simulink model "ALL_JP360_DBW_V6_5_1103"  (R2022a)
settings: Solver=FixedStepAuto  StartTime=0.0  StopTime=inf  FixedStep=0.01  RelTol=1e-3  EnableMultiTasking=on
model workspace (MAT data in the model file):
  g = 9.8
undefined symbols (not defined in the file or in its folder): canChannel, delta_v_p, IPM_Line_C0, IPM_Line_C1, IPM_Line_C2, IPM_Line_C3, M, M_p, MRR_ObjDistX, MRR_ObjDistY, MRR_ObjFusionCamID, MRR_ObjFusionSig, MRR_ObjID, MRR_ObjRelVelX, MRR_ObjRelVelY, MRR_ObjType, MRR_ObjUpdFlg, none, obj_vaild, untracktime, V, videoinput
libraries: canfdmsglib x230, canfdlib x76, slpidlib x24, simulink x18, dspstat3 x14, ctrlSharedLib x1, simulink_extras x1, imaqlib x1, realtime_pacer_lib x1, dspvision x1, visionsinks x1
(part 3 of 55)

== system ALL_JP360_DBW_V6_5_1103/MsgToCAN ==
  ACC_Torque_Request : Inport
  ACC_Torque_Request_Status : Inport  Port=2
  ACC_TgtAx : Inport  Port=3
  ACC_BrakePreferred : Inport  Port=4
  ACC_StandstillReq : Inport  Port=5
  ACC_Status : Inport  Port=6
  setvspped : Inport  Port=7
  ACC_TimeGapSet : Inport  Port=8
  ACC_EngineStartstop : Inport  Port=9
  IPM_LaneAssit_Status : Inport  Port=10
  IPM_LaneAssit_TorqueReq : Inport  Port=11
  IPM_LaneAssit_TorqueReqStatus : Inport  Port=12
  Obj_Speed : Inport  Port=13
  ACC_ObjDetected : Inport  Port=14
  MRR_L_Obj_0x_class : Inport  Port=15
  MRR_L_Object_dx : Inport  Port=16
  MRR_L_Object_dy : Inport  Port=17
  MRR_LeftTargetDetection : Inport  Port=18
  MRR_R_Obj_0x_class : Inport  Port=19
  MRR_R_Object_dx : Inport  Port=20
  MRR_R_Object_dy : Inport  Port=21
  MRR_RightTargetDetection : Inport  Port=22
  MRR_F_Object_dx : Inport  Port=23
  MRR_F_Object_dy : Inport  Port=24
  MRR_F_Obj_0x_class : Inport  Port=25
  640 : Inport  Port=26
  641 : Inport  Port=27
  642 : Inport  Port=28
  643 : Inport  Port=29
  ACC_DriveOff : Inport  Port=30
  CAN FD Transmit1 : canfdlib/CAN FD Transmit  BlockHandle=28204.001  Device=Vector VN1640A 1 (Channel 3)  ObjConstructor=canChannel('Vector', 'VN1640A 1', 3, 'ProtocolMode', 'CAN FD')  EnableEventTransmit=off  EnablePeriodicTransmit=on  MessagePeriod=0.02
      settings: SourceProductBaseCode=VN
  CAN FD Transmit10 : canfdlib/CAN FD Transmit  BlockHandle=28206.001  Device=Vector VN1640A 1 (Channel 3)  ObjConstructor=canChannel('Vector', 'VN1640A 1', 3, 'ProtocolMode', 'CAN FD')  EnableEventTransmit=off  EnablePeriodicTransmit=on  MessagePeriod=0.1
      settings: SourceProductBaseCode=VN
  CAN FD Transmit11 : canfdlib/CAN FD Transmit  BlockHandle=28208.001  Device=Vector VN1640A 1 (Channel 3)  ObjConstructor=canChannel('Vector', 'VN1640A 1', 3, 'ProtocolMode', 'CAN FD')  EnableEventTransmit=off  EnablePeriodicTransmit=on  MessagePeriod=0.1
      settings: SourceProductBaseCode=VN
  CAN FD Transmit2 : canfdlib/CAN FD Transmit  BlockHandle=28210.001  Device=Vector VN1640A 1 (Channel 3)  ObjConstructor=canChannel('Vector', 'VN1640A 1', 3, 'ProtocolMode', 'CAN FD')  EnableEventTransmit=off  EnablePeriodicTransmit=on  MessagePeriod=0.02
      settings: SourceProductBaseCode=VN
  CAN FD Transmit3 : canfdlib/CAN FD Transmit  BlockHandle=28212.001  Device=Vector VN1640A 1 (Channel 3)  ObjConstructor=canChannel('Vector', 'VN1640A 1', 3, 'ProtocolMode', 'CAN FD')  EnableEventTransmit=off  EnablePeriodicTransmit=on  MessagePeriod=0.02
      settings: SourceProductBaseCode=VN
  CAN FD Transmit4 : canfdlib/CAN FD Transmit  BlockHandle=28214.001  Device=Vector VN1640A 1 (Channel 3)  ObjConstructor=canChannel('Vector', 'VN1640A 1', 3, 'ProtocolMode', 'CAN FD')  EnableEventTransmit=off  EnablePeriodicTransmit=on  MessagePeriod=0.02
      settings: SourceProductBaseCode=VN
  CAN FD Transmit5 : canfdlib/CAN FD Transmit  BlockHandle=28216.001  Device=Vector VN1640A 1 (Channel 3)  ObjConstructor=canChannel('Vector', 'VN1640A 1', 3, 'ProtocolMode', 'CAN FD')  EnableEventTransmit=off  EnablePeriodicTransmit=on  MessagePeriod=0.02
      settings: SourceProductBaseCode=VN
  CAN FD Transmit6 : canfdlib/CAN FD Transmit  BlockHandle=28218.001  Device=Vector VN1640A 1 (Channel 3)  ObjConstructor=canChannel('Vector', 'VN1640A 1', 3, 'ProtocolMode', 'CAN FD')  EnableEventTransmit=off  EnablePeriodicTransmit=on  MessagePeriod=0.02
      settings: SourceProductBaseCode=VN
  CAN FD Transmit7 : canfdlib/CAN FD Transmit  BlockHandle=28220.001  Device=Vector VN1640A 1 (Channel 3)  ObjConstructor=canChannel('Vector', 'VN1640A 1', 3, 'ProtocolMode', 'CAN FD')  EnableEventTransmit=off  EnablePeriodicTransmit=on  MessagePeriod=0.02
      settings: SourceProductBaseCode=VN
  CAN FD Transmit8 : canfdlib/CAN FD Transmit  BlockHandle=28222.001  Device=Vector VN1640A 1 (Channel 3)  ObjConstructor=canChannel('Vector', 'VN1640A 1', 3, 'ProtocolMode', 'CAN FD')  EnableEventTransmit=off  EnablePeriodicTransmit=on  MessagePeriod=0.1
      settings: SourceProductBaseCode=VN
  CAN FD Transmit9 : canfdlib/CAN FD Transmit  BlockHandle=28224.001  Device=Vector VN1640A 1 (Channel 3)  ObjConstructor=canChannel('Vector', 'VN1640A 1', 3, 'ProtocolMode', 'CAN FD')  EnableEventTransmit=off  EnablePeriodicTransmit=on  MessagePeriod=0.1
      settings: SourceProductBaseCode=VN
  CCAN_ADCU_MsgFromCAN : Subsystem
  CCAN_ADCU_MsgToCAN : Subsystem
  wires:
  CCAN_ADCU_MsgFromCAN/11(CCAN_ADCU_MRR_0x238FromOutData) -> CCAN_ADCU_MsgToCAN/11(CCAN_ADCU_MRR_0x238ToInData)  "CCAN_ADCU_MRR_0x238FromOutData"
  CCAN_ADCU_MsgFromCAN/13(CCAN_ADCU_MRR_0x246FromOutData) -> CCAN_ADCU_MsgToCAN/13(CCAN_ADCU_MRR_0x246ToInData)  "CCAN_ADCU_MRR_0x246FromOutData"
  CCAN_ADCU_MsgFromCAN/15(CCAN_ADCU_MRR_LRObj_0x480FromOutData) -> CCAN_ADCU_MsgToCAN/15(CCAN_ADCU_MRR_LRObj_0x480ToInData)  "CCAN_ADCU_MRR_LRObj_0x480FromOutData"
  CCAN_ADCU_MsgToCAN/7(CCAN_ADCU_IPM_LeftLine_0x280ToOutData) -> CAN FD Transmit11/1  "CCAN_ADCU_IPM_LeftLine_0x280ToOutData"
  CCAN_ADCU_MsgToCAN/9(CCAN_ADCU_IPM_RightLine_0x491ToOutData) -> CAN FD Transmit10/1  "CCAN_ADCU_IPM_RightLine_0x491ToOutData"
  CCAN_ADCU_MsgToCAN/11(CCAN_ADCU_MRR_0x238ToOutData) -> CAN FD Transmit5/1  "CCAN_ADCU_MRR_0x238ToOutData"
  CCAN_ADCU_MsgFromCAN/12(CCAN_ADCU_MRR_0x239FromOutData) -> CCAN_ADCU_MsgToCAN/12(CCAN_ADCU_MRR_0x239ToInData)  "CCAN_ADCU_MRR_0x239FromOutData"
  CCAN_ADCU_MsgFromCAN/14(CCAN_ADCU_MRR_FRObj_0x279FromOutData) -> CCAN_ADCU_MsgToCAN/14(CCAN_ADCU_MRR_FRObj_0x279ToInData)  "CCAN_ADCU_MRR_FRObj_0x279FromOutData"
  CCAN_ADCU_MsgFromCAN/16(CCAN_ADCU_TIMESYNC_analy_620FromOutData) -> CCAN_ADCU_MsgToCAN/16(CCAN_ADCU_TIMESYNC_analy_620ToInData)  "CCAN_ADCU_TIMESYNC_analy_620FromOutData"
  ACC_StandstillReq/1 -> CCAN_ADCU_MsgFromCAN/5(ACC_StandstillReq)
  CCAN_ADCU_MsgToCAN/6(CCAN_ADCU_IPM_LeftLine_0x278ToOutData) -> CAN FD Transmit8/1  "CCAN_ADCU_IPM_LeftLine_0x278ToOutData"
  CCAN_ADCU_MsgToCAN/10(CCAN_ADCU_IPM_VLC_0x293ToOutData) -> CAN FD Transmit1/1  "CCAN_ADCU_IPM_VLC_0x293ToOutData"
  CCAN_ADCU_MsgToCAN/8(CCAN_ADCU_IPM_RightLine_0x490ToOutData) -> CAN FD Transmit9/1  "CCAN_ADCU_IPM_RightLine_0x490ToOutData"
  CCAN_ADCU_MsgToCAN/4(CCAN_ADCU_IPM_0x245ToOutData) -> CAN FD Transmit2/1  "CCAN_ADCU_IPM_0x245ToOutData"
  CCAN_ADCU_MsgToCAN/15(CCAN_ADCU_MRR_LRObj_0x480ToOutData) -> CAN FD Transmit7/1  "CCAN_ADCU_MRR_LRObj_0x480ToOutData"
  CCAN_ADCU_MsgToCAN/13(CCAN_ADCU_MRR_0x246ToOutData) -> CAN FD Transmit4/1
  CCAN_ADCU_MsgToCAN/14(CCAN_ADCU_MRR_FRObj_0x279ToOutData) -> CAN FD Transmit6/1  "CCAN_ADCU_MRR_FRObj_0x279ToOutData"
  CCAN_ADCU_MsgToCAN/12(CCAN_ADCU_MRR_0x239ToOutData) -> CAN FD Transmit3/1  "CCAN_ADCU_MRR_0x239ToOutData"
  ACC_DriveOff/1 -> CCAN_ADCU_MsgFromCAN/30(ACC_DriveOff)
  CCAN_ADCU_MsgFromCAN/2(CCAN_ADCU_ADCU_CanTSyn_0x570FromOutData) -> CCAN_ADCU_MsgToCAN/2(CCAN_ADCU_ADCU_CanTSyn_0x570ToInData)  "CCAN_ADCU_ADCU_CanTSyn_0x570FromOutData"
  ACC_TgtAx/1 -> CCAN_ADCU_MsgFromCAN/3(ACC_TgtAx)
  Obj_Speed/1 -> CCAN_ADCU_MsgFromCAN/13(Obj_Speed)
  MRR_R_Obj_0x_class/1 -> CCAN_ADCU_MsgFromCAN/19(MRR_R_Obj_0x_class)
  MRR_F_Obj_0x_class/1 -> CCAN_ADCU_MsgFromCAN/25(MRR_F_Obj_0x_class)
  MRR_F_Object_dy/1 -> CCAN_ADCU_MsgFromCAN/24(MRR_F_Object_dy)
  CCAN_ADCU_MsgFromCAN/1(CCAN_ADCU_ADCU_0x538FromOutData) -> CCAN_ADCU_MsgToCAN/1(CCAN_ADCU_ADCU_0x538ToInData)  "CCAN_ADCU_ADCU_0x538FromOutData"
  ACC_EngineStartstop/1 -> CCAN_ADCU_MsgFromCAN/9(ACC_EngineStartstop)
  MRR_RightTargetDetection/1 -> CCAN_ADCU_MsgFromCAN/22(MRR_RightTargetDetection)
  MRR_L_Obj_0x_class/1 -> CCAN_ADCU_MsgFromCAN/15(MRR_L_Obj_0x_class)
  MRR_F_Object_dx/1 -> CCAN_ADCU_MsgFromCAN/23(MRR_F_Object_dx)
  MRR_L_Object_dx/1 -> CCAN_ADCU_MsgFromCAN/16(MRR_L_Object_dx)
  ACC_BrakePreferred/1 -> CCAN_ADCU_MsgFromCAN/4(ACC_BrakePreferred)
  ACC_ObjDetected/1 -> CCAN_ADCU_MsgFromCAN/14(ACC_ObjDetected)
  MRR_R_Object_dy/1 -> CCAN_ADCU_MsgFromCAN/21(MRR_R_Object_dy)
  MRR_L_Object_dy/1 -> CCAN_ADCU_MsgFromCAN/17(MRR_L_Object_dy)
  MRR_R_Object_dx/1 -> CCAN_ADCU_MsgFromCAN/20(MRR_R_Object_dx)
  643/1 -> CCAN_ADCU_MsgFromCAN/29(643)
  642/1 -> CCAN_ADCU_MsgFromCAN/28(642)
  641/1 -> CCAN_ADCU_MsgFromCAN/27(641)
  IPM_LaneAssit_TorqueReq/1 -> CCAN_ADCU_MsgFromCAN/11(IPM_LaneAssit_TorqueReq)
  640/1 -> CCAN_ADCU_MsgFromCAN/26(640)
  ACC_Torque_Request_Status/1 -> CCAN_ADCU_MsgFromCAN/2(ACC_Torque_Request_Status)
  IPM_LaneAssit_Status/1 -> CCAN_ADCU_MsgFromCAN/10(IPM_LaneAssit_Status)
  MRR_LeftTargetDetection/1 -> CCAN_ADCU_MsgFromCAN/18(MRR_LeftTargetDetection)
  IPM_LaneAssit_TorqueReqStatus/1 -> CCAN_ADCU_MsgFromCAN/12(IPM_LaneAssit_TorqueReqStatus)
  ACC_TimeGapSet/1 -> CCAN_ADCU_MsgFromCAN/8(ACC_TimeGapSet)
  setvspped/1 -> CCAN_ADCU_MsgFromCAN/7(setvspped)
  ACC_Status/1 -> CCAN_ADCU_MsgFromCAN/6(ACC_Status)
  ACC_Torque_Request/1 -> CCAN_ADCU_MsgFromCAN/1(ACC_Torque_Request)
  CCAN_ADCU_MsgFromCAN/4(CCAN_ADCU_IPM_0x245FromOutData) -> CCAN_ADCU_MsgToCAN/4(CCAN_ADCU_IPM_0x245ToInData)  "CCAN_ADCU_IPM_0x245FromOutData"
  CCAN_ADCU_MsgFromCAN/6(CCAN_ADCU_IPM_LeftLine_0x278FromOutData) -> CCAN_ADCU_MsgToCAN/6(CCAN_ADCU_IPM_LeftLine_0x278ToInData)  "CCAN_ADCU_IPM_LeftLine_0x278FromOutData"
  CCAN_ADCU_MsgFromCAN/8(CCAN_ADCU_IPM_RightLine_0x490FromOutData) -> CCAN_ADCU_MsgToCAN/8(CCAN_ADCU_IPM_RightLine_0x490ToInData)  "CCAN_ADCU_IPM_RightLine_0x490FromOutData"
  CCAN_ADCU_MsgFromCAN/10(CCAN_ADCU_IPM_VLC_0x293FromOutData) -> CCAN_ADCU_MsgToCAN/10(CCAN_ADCU_IPM_VLC_0x293ToInData)  "CCAN_ADCU_IPM_VLC_0x293FromOutData"
  CCAN_ADCU_MsgFromCAN/3(CCAN_ADCU_ADCU_DiagRespFromOutData) -> CCAN_ADCU_MsgToCAN/3(CCAN_ADCU_ADCU_DiagRespToInData)  "CCAN_ADCU_ADCU_DiagRespFromOutData"
  CCAN_ADCU_MsgFromCAN/5(CCAN_ADCU_IPM_0x247FromOutData) -> CCAN_ADCU_MsgToCAN/5(CCAN_ADCU_IPM_0x247ToInData)  "CCAN_ADCU_IPM_0x247FromOutData"
  CCAN_ADCU_MsgFromCAN/7(CCAN_ADCU_IPM_LeftLine_0x280FromOutData) -> CCAN_ADCU_MsgToCAN/7(CCAN_ADCU_IPM_LeftLine_0x280ToInData)  "CCAN_ADCU_IPM_LeftLine_0x280FromOutData"
  CCAN_ADCU_MsgFromCAN/9(CCAN_ADCU_IPM_RightLine_0x491FromOutData) -> CCAN_ADCU_MsgToCAN/9(CCAN_ADCU_IPM_RightLine_0x491ToInData)  "CCAN_ADCU_IPM_RightLine_0x491FromOutData"

== system ALL_JP360_DBW_V6_5_1103/Subsystem1 ==
  LKAReq_angle : Inport
  IPM_LineAssit_Status : Inport  Port=2
  DCLC_status : Inport  Port=3  OutDataTypeStr=int16
  DCLCRequestTorque : Inport  Port=4
  Constant1 : Constant  Value=4  OutDataTypeStr=int8
  Constant6 : Constant  Value=0  OutDataTypeStr=single
  Display{,1..5} (6 alike) : Display
  Equal : RelationalOperator  Operator===  OutDataTypeStr=boolean  RndMeth=Simplest  InputSameDT=off
  Scope : Scope  NumInputPorts=4
  Switch : Switch  Criteria=u2 ~= 0  OutDataTypeStr=single  SaturateOnIntegerOverflow=off  InputSameDT=off
  Switch1 : Switch  Threshold=2  OutDataTypeStr=single  SaturateOnIntegerOverflow=off  InputSameDT=off
  torque_req : Outport
  wires:
  DCLC_status/1 -> Scope/4, Switch1/2, Display1/1  "dclc_status"
  Switch/1 -> Display3/1, Scope/3, Switch1/3  "lka_req"
  Constant6/1 -> Switch/3
  LKAReq_angle/1 -> Display4/1, Switch/1
  Switch1/1 -> Scope/1, torque_req/1, Display/1  "req_out"
  DCLCRequestTorque/1 -> Scope/2, Switch1/1, Display5/1  "dclc_req"
  IPM_LineAssit_Status/1 -> Equal/1
  Constant1/1 -> Equal/2
  Equal/1 -> Display2/1, Switch/2

== system ALL_JP360_DBW_V6_5_1103/button ==
  SWM_ACCSwitch : Inport
  TimeGapSet : Inport  Port=2
  SWM_ACCvSetPlus : Inport  Port=3
  SWM_ACCvSetMinus : Inport  Port=4
  acc_status : Inport  Port=5
  set_speed_out : Inport  Port=6
  ACCset : Subsystem
  Constant : Constant  Value=3  OutDataTypeStr=int8
  Manual Switch : ManualSwitch
  TimeGapSetOut : Outport
  setvspeed : Outport  Port=2
  Out3 : Outport  Port=3
  wires:
  Manual Switch/1 -> ACCset/2(acc_status)
  SWM_ACCvSetMinus/1 -> ACCset/6(SWM_ACCvSetMinus)
  SWM_ACCvSetPlus/1 -> ACCset/5(SWM_ACCvSetPlus)
  ACCset/3(Out3) -> Out3/1
  TimeGapSet/1 -> ACCset/4(TimeGapSet)
  ACCset/1(setvspeed) -> setvspeed/1
  ACCset/2(TimeGapSetOut) -> TimeGapSetOut/1
  SWM_ACCSwitch/1 -> ACCset/1(SWM_ACCSwitch)
  set_speed_out/1 -> ACCset/3(set_speed_out)
  acc_status/1 -> Manual Switch/1
  Constant/1 -> Manual Switch/2

== system ALL_JP360_DBW_V6_5_1103/ACC_Control/ACC_FUNCTION ==
  Ego_speed : Inport
  SWM_ACCSwitch : Inport  Port=2
  SWM_ACCSet : Inport  Port=3
  SWM_ACCResume : Inport  Port=4
  BCM_DoorStsFrntLe : Inport  Port=5
  BCM_DoorStsFrntRi : Inport  Port=6
  BCM_DoorStsRearLe : Inport  Port=7
  BCM_DoorStsRearRi : Inport  Port=8
  IPM_SensorState : Inport  Port=9
  MRR_HWFail : Inport  Port=10
  BCM_PowerModeInvalid : Inport  Port=11
  BCM_PowerMode : Inport  Port=12
  BCM_Mechanical_Hand_Brake : Inport  Port=13
  BCM_EnginehoodSts : Inport  Port=14
  SRS_SBR_Driver : Inport  Port=15
  EMS_IndicatedEngError : Inport  Port=16
  EMS_AccRAWPedalRatio : Inport  Port=17
  EMS_BrkPedalStasus : Inport  Port=18
  EPS_EPSPAMSts : Inport  Port=19
  TCU_GearSelectorReq : Inport  Port=20
  ESP_EPBStatus : Inport  Port=21
  ESP_EspEnableSts : Inport  Port=22
  ABS_VehSpdDirection : Inport  Port=23
  ESP_AvhActive : Inport  Port=24
  ESP_VehicleStandstill : Inport  Port=25
  HWT_dem[s] : Inport  Port=26
  Des_speed[km/h] : Inport  Port=27
  CIPV_detected_flag : Inport  Port=28
  CIPV_distance : Inport  Port=29
  CIPV_velocity : Inport  Port=30
  EMS_IndicatedDriverOverride : Inport  Port=31
  set_speed_in : Inport  Port=32
  ax_esp : Inport  Port=33
  ay_esp : Inport  Port=34
  yaw_rate : Inport  Port=35
  steer_angle : Inport  Port=36
  IC_VehSpd_HMI : Inport  Port=37
  Add : Sum  Inputs=+-
  Add1 : Sum
  Constant : Constant  Value=0  OutDataTypeStr=boolean  SampleTime=-1
  Constant1 : Constant  Value=0.5  OutDataTypeStr=single
  Constant2 : Constant  Value=3  OutDataTypeStr=int8
  Constant3 : Constant  Value=0  OutDataTypeStr=int8
  Constant4 : Constant  OutDataTypeStr=int8
  Constant5 : Constant  Value=0.5  OutDataTypeStr=single
  Data Type Conversion1 : DataTypeConversion  OutDataTypeStr=single  SaturateOnIntegerOverflow=off  RndMeth=Floor
  Product : Product
  Product1 : Product
  Saturation : Saturate  UpperLimit=150  LowerLimit=0
  Saturation1 : Saturate  UpperLimit=150  LowerLimit=0
  Saturation2 : Saturate  UpperLimit=50  LowerLimit=-50
  Scope : Scope
  Subsystem2 : Subsystem  mask{mass=2200, Width=2.165, Hight=1.871, C_d=0.35, C_f0=0.015, C_fk=0.0002, r_tire=0.34, thgma_total=1.06, Standstill_distance=4, Moving_Average_Window=6, slope_threshold=1.2, kph2mps=1/3.6}
      mask prompts: mass "整车质量mass"; Width "整车宽度Width"; Hight "整车高度Hight"; C_d "风阻系数C_d"; C_f0 "滚动阻力系数初值C_f0"; C_fk "滚动阻力系数随速度变化率C_fk"; r_tire "轮胎半径r_tire"; thgma_total "质量转换系数thgma_total"; Standstill_distance "最小安全距离Standstill_distance"; Moving_Average_Window "加速度滤波窗口长度"; slope_threshold "坡度阈值"; kph2mps "km/h转换到m/s"
      mask DialogControl ParameterGroupVar Prompt: 参数
  Switch : Switch  Criteria=u2 ~= 0  SaturateOnIntegerOverflow=off  InputSameDT=off
  acc_stateflow : Subsystem
  acc_status : Outport
  acc_torque[NM] : Outport  Port=2
  acc_brake[ms-2] : Outport  Port=3
  set_speed_out : Outport  Port=4
  standstill_req : Outport  Port=5
  ACC_DriveOff : Outport  Port=6
  wires:
  Ego_speed/1 -> [Ego_speed]
  Product/1 -> Saturation/1
  acc_stateflow/1(ACC_Status) -> Subsystem2/1(Acc_status), Add/1, acc_status/1
  EMS_IndicatedDriverOverride/1 -> acc_stateflow/26(EMS_IndicatedDriverOverride)
  [IC_VehSpd_HMI] -> acc_stateflow/27(ABS_VehSpdLgt)
  set_speed_in/1 -> acc_stateflow/28(set_speed_in)
  acc_stateflow/2(set_speed_out) -> Scope/1, set_speed_out/1
  IC_VehSpd_HMI/1 -> [IC_VehSpd_HMI], Data Type Conversion1/1
  Constant2/1 -> Add/2
  Add/1 -> Switch/2
  Constant3/1 -> Switch/1
  Constant4/1 -> Switch/3
  Switch/1 -> Product/1
  Des_speed[km/h]/1 -> [Des_speed_kph], Product/2
  Subsystem2/2(acc_throttle [nm]) -> acc_torque[NM]/1
  Subsystem2/1(standstill_req) -> standstill_req/1
  Subsystem2/3(acc_brake [-a]) -> acc_brake[ms-2]/1
  Saturation/1 -> Subsystem2/12(Set_speed_kph[km/h])
  ax_esp/1 -> Subsystem2/8(ax_esp [m/s2])
  ay_esp/1 -> Subsystem2/9(ay_esp[m/s2])
  yaw_rate/1 -> Subsystem2/10(yaw_rate[deg/s])
  steer_angle/1 -> Subsystem2/11(steer_angle[deg])
  [CIPV_detected_flag] -> Subsystem2/7(obj_detacted_flag)
  CIPV_distance/1 -> Saturation1/1
  Data Type Conversion1/1 -> Subsystem2/3(Ego_velocity_IC [km/h])
  [Ego_speed] -> Subsystem2/2(Ego_velocity_abs [km/h])
  CIPV_velocity/1 -> Saturation2/1
  [cipv_x] -> acc_stateflow/31(CIPV_ObjDistX)
  Constant/1 -> acc_stateflow/25(acc_state_sw)
  [cipv_s] -> acc_stateflow/30(Obj_Speed)
  ESP_VehicleStandstill/1 -> acc_stateflow/24(ESP_VehicleStandstill)
  ESP_AvhActive/1 -> acc_stateflow/23(ESP_AvhActive)
  ABS_VehSpdDirection/1 -> acc_stateflow/22(ABS_VehSpdDirection)
  ESP_EspEnableSts/1 -> acc_stateflow/21(ESP_EspEnableSts)
  ESP_EPBStatus/1 -> acc_stateflow/20(ESP_EPBStatus)
  TCU_GearSelectorReq/1 -> acc_stateflow/19(TCU_GearSelectorReq)
  EPS_EPSPAMSts/1 -> acc_stateflow/18(EPS_EPSPAMSts)
  EMS_BrkPedalStasus/1 -> acc_stateflow/17(EMS_BrkPedalStasus)
  EMS_AccRAWPedalRatio/1 -> acc_stateflow/16(EMS_AccRAWPedalRatio)
  EMS_IndicatedEngError/1 -> acc_stateflow/15(EMS_IndicatedEngError)
  SRS_SBR_Driver/1 -> acc_stateflow/14(SRS_SBR_Driver)
  MRR_HWFail/1 -> acc_stateflow/13(MRR_HWFail)
  IPM_SensorState/1 -> acc_stateflow/12(IPM_SensorState)
  BCM_EnginehoodSts/1 -> acc_stateflow/11(BCM_EnginehoodSts)
  BCM_Mechanical_Hand_Brake/1 -> acc_stateflow/10(BCM_Mechanical_Hand_Brake)
  BCM_PowerMode/1 -> acc_stateflow/9(BCM_PowerMode)
  BCM_PowerModeInvalid/1 -> acc_stateflow/8(BCM_PowerModeInvalid)
  BCM_DoorStsRearRi/1 -> acc_stateflow/7(BCM_DoorStsRearRi)
  BCM_DoorStsRearLe/1 -> acc_stateflow/6(BCM_DoorStsRearLe)
  BCM_DoorStsFrntRi/1 -> acc_stateflow/5(BCM_DoorStsFrntRi)
  BCM_DoorStsFrntLe/1 -> acc_stateflow/4(BCM_DoorStsFrntLe)
  SWM_ACCResume/1 -> acc_stateflow/3(SWM_ACCResume)
  SWM_ACCSet/1 -> acc_stateflow/2(SWM_ACCSet)
  SWM_ACCSwitch/1 -> acc_stateflow/1(SWM_ACCSwitch)
  acc_stateflow/3(ACC_DriveOff) -> ACC_DriveOff/1
  CIPV_detected_flag/1 -> [CIPV_detected_flag], acc_stateflow/29(ACC_ObjDetected)
  HWT_dem[s]/1 -> Product1/2
  Constant1/1 -> Product1/1
  Product1/1 -> Add1/1
  Constant5/1 -> Add1/2
  Add1/1 -> Subsystem2/6(HWT_dem [s])
  Saturation1/1 -> [cipv_x], Subsystem2/4(TIS1_range [m])
  Saturation2/1 -> Subsystem2/5(TIS1_rangedot [m/s]), [cipv_s]

== system ALL_JP360_DBW_V6_5_1103/CIPV1/Lane Line Construction1 ==
  IPM_Line_left : Inport
  IPM_Line_right : Inport  Port=2
  IPM_Line_left_left : Inport  Port=3
  IPM_Line_right_right : Inport  Port=4
  SAS_SteerWheelAngle : Inport  Port=5
  EGO_yaw_rate : Inport  Port=6
  EGO_speed : Inport  Port=7
  Abs : Abs  SaturateOnIntegerOverflow=off
  Bus Creator{,1..3} (4 alike) : BusCreator  Inputs=IPM_Line_C0,IPM_Line_C1,IPM_Line_C2,IPM_Line_C3
  Bus Selector1 : BusSelector  OutputSignals=IPM_Line02_Existence_Probability,IPM_Line02_Type,IPM_Line02_C0,IPM_Line02_C1,IPM_Line02_C2,IPM_Line02_C3
  Bus Selector10 : BusSelector  OutputSignals=IPM_Line01_Existence_Probability,IPM_Line01_Type,IPM_Line01_C0,IPM_Line01_C1,IPM_Line01_C2,IPM_Line01_C3
  Bus Selector2 : BusSelector  OutputSignals=IPM_Line03_Existence_Probability,IPM_Line03_C0,IPM_Line03_C1,IPM_Line03_C2,IPM_Line03_C3
  Bus Selector3 : BusSelector  OutputSignals=IPM_Line04_Existence_Probability,IPM_Line04_C0,IPM_Line04_C1,IPM_Line04_C2,IPM_Line04_C3
  Degrees to Radians : simulink_extras/Transformations/Degrees to Radians
  Demux{,1..3} (4 alike) : Demux
  Divide1 : Product  Inputs=*/
  Divide2 : Product  Inputs=*/
  Embedded MATLAB Function1 : MATLAB Function  TreatAsAtomicUnit=on
  Embedded MATLAB Function10 : MATLAB Function  TreatAsAtomicUnit=on
  Embedded MATLAB Function2 : MATLAB Function  TreatAsAtomicUnit=on
  Embedded MATLAB Function3 : MATLAB Function  TreatAsAtomicUnit=on
  Embedded MATLAB Function4 : MATLAB Function  TreatAsAtomicUnit=on
  Embedded MATLAB Function5 : MATLAB Function  TreatAsAtomicUnit=on
  Embedded MATLAB Function6 : MATLAB Function  TreatAsAtomicUnit=on
  Embedded MATLAB Function7 : MATLAB Function  TreatAsAtomicUnit=on
  Embedded MATLAB Function8 : MATLAB Function  TreatAsAtomicUnit=on
  Embedded MATLAB Function9 : MATLAB Function  TreatAsAtomicUnit=on
  Switch{1..4} (4 alike) : Switch  Criteria=u2 ~= 0  SaturateOnIntegerOverflow=off  InputSameDT=off
  steering ratio : Constant  Value=17.2  OutDataTypeStr=int8
  wheelbase : Constant  Value=3.27  OutDataTypeStr=int8
  left_line : Outport
  right_line : Outport  Port=2
  left_left_line : Outport  Port=3
  right_right_line : Outport  Port=4
  wires:
  Embedded MATLAB Function7/1(judge) -> Switch4/2
  Divide2/1 -> Abs/1
  Embedded MATLAB Function8/1(line_data) -> Switch4/3
  Embedded MATLAB Function5/1(judge) -> Switch3/2
  Embedded MATLAB Function2/1(judge) -> Switch1/2
  Switch4/1 -> Demux3/1
  Embedded MATLAB Function4/1(judge) -> Switch2/2
  Embedded MATLAB Function2/2(line_data) -> Switch1/1
  Bus Creator/1 -> left_line/1
  Demux3/2 -> Bus Creator3/2  "IPM_Line_C1"
  Switch2/1 -> Demux1/1
  Bus Selector1/6 -> Embedded MATLAB Function10/5(IPM_Line_C3), Embedded MATLAB Function4/5(IPM_Line_C3)  "<IPM_Line02_C3>"
  Bus Selector1/5 -> Embedded MATLAB Function4/4(IPM_Line_C2), Embedded MATLAB Function10/4(IPM_Line_C2)  "<IPM_Line02_C2>"
  Bus Creator3/1 -> right_right_line/1
  Bus Selector10/1 -> Embedded MATLAB Function9/1(IPM_Line_Existence_Probability), Embedded MATLAB Function2/1(IPM_Line_Existence_Probability)  "<IPM_Line01_Existence_Probability>"
  Demux2/3 -> Bus Creator2/3  "IPM_Line_C2"
  Bus Selector10/5 -> Embedded MATLAB Function9/4(IPM_Line_C2), Embedded MATLAB Function2/4(IPM_Line_C2)  "<IPM_Line01_C2>"
  Bus Selector1/3 -> Embedded MATLAB Function10/2(IPM_Line_C0), Embedded MATLAB Function4/2(IPM_Line_C0)  "<IPM_Line02_C0>"
  Bus Selector3/1 -> Embedded MATLAB Function7/2(IPM_Line_Existence_Probability)  "<IPM_Line04_Existence_Probability>"
  Demux2/2 -> Bus Creator2/2  "IPM_Line_C1"
  Bus Creator1/1 -> right_line/1
  Divide1/1 -> Divide2/2
  Demux3/4 -> Bus Creator3/4  "IPM_Line_C3"
  Switch3/1 -> Demux2/1
  Bus Selector1/4 -> Embedded MATLAB Function4/3(IPM_Line_C1), Embedded MATLAB Function10/3(IPM_Line_C1)  "<IPM_Line02_C1>"
  Demux2/1 -> Bus Creator2/1  "IPM_Line_C0"
  Embedded MATLAB Function7/2(line_data) -> Switch4/1
  Demux3/3 -> Bus Creator3/3  "IPM_Line_C2"
  Demux1/4 -> Bus Creator1/4  "IPM_Line_C3"
  Bus Selector3/2 -> Embedded MATLAB Function7/3(IPM_Line_C0)  "<IPM_Line04_C0>"
  Bus Creator2/1 -> left_left_line/1
  Demux1/1 -> Bus Creator1/1  "IPM_Line_C0"
  Embedded MATLAB Function3/1(line_data) -> Switch2/3
  IPM_Line_left/1 -> Bus Selector10/1
  Demux2/4 -> Bus Creator2/4  "IPM_Line_C3"
  Embedded MATLAB Function4/2(line_data) -> Switch2/1
  Demux/1 -> Bus Creator/1  "IPM_Line_C0"
  steering ratio/1 -> Divide1/2
  Demux1/2 -> Bus Creator1/2  "IPM_Line_C1"
  Demux/4 -> Bus Creator/4  "IPM_Line_C3"
  Switch1/1 -> Demux/1
  Bus Selector1/2 -> Embedded MATLAB Function8/3(IPM_Line_type), Embedded MATLAB Function7/1(IPM_Line_type)  "<IPM_Line02_Type>"
  Embedded MATLAB Function9/1(judge_cover_line) -> Embedded MATLAB Function7/7(judge_cover_line_left), Embedded MATLAB Function5/7(judge_cover_line_left), Embedded MATLAB Function4/6(judge_cover_line_left), Embedded MATLAB Function2/6(judge_cover_line_left)
  IPM_Line_left_left/1 -> Bus Selector2/1
  Demux/2 -> Bus Creator/2  "IPM_Line_C1"
  wheelbase/1 -> Divide2/1
  Embedded MATLAB Function10/1(judge_cover_line) -> Embedded MATLAB Function2/7(judge_cover_line_right), Embedded MATLAB Function7/8(judge_cover_line_right), Embedded MATLAB Function5/8(judge_cover_line_right), Embedded MATLAB Function4/7(judge_cover_line_right)
  SAS_SteerWheelAngle/1 -> Degrees to Radians/1, Embedded MATLAB Function8/2(SteerWheelAngle), Embedded MATLAB Function1/2(SteerWheelAngle), Embedded MATLAB Function3/2(SteerWheelAngle), Embedded MATLAB Function6/2(SteerWheelAngle)
  Demux3/1 -> Bus Creator3/1  "IPM_Line_C0"
  Bus Selector2/2 -> Embedded MATLAB Function5/3(IPM_Line_C0)  "<IPM_Line03_C0>"
  Abs/1 -> Embedded MATLAB Function8/1(R), Embedded MATLAB Function6/1(R), Embedded MATLAB Function3/1(R), Embedded MATLAB Function1/1(R)
  Bus Selector1/1 -> Embedded MATLAB Function10/1(IPM_Line_Existence_Probability), Embedded MATLAB Function4/1(IPM_Line_Existence_Probability)  "<IPM_Line02_Existence_Probability>"
  Bus Selector2/3 -> Embedded MATLAB Function5/4(IPM_Line_C1)  "<IPM_Line03_C1>"
  Bus Selector3/4 -> Embedded MATLAB Function7/5(IPM_Line_C2)  "<IPM_Line04_C2>"
  Bus Selector2/1 -> Embedded MATLAB Function5/2(IPM_Line_Existence_Probability)  "<IPM_Line03_Existence_Probability>"
  Bus Selector3/3 -> Embedded MATLAB Function7/4(IPM_Line_C1)  "<IPM_Line04_C1>"
  Bus Selector10/6 -> Embedded MATLAB Function9/5(IPM_Line_C3), Embedded MATLAB Function2/5(IPM_Line_C3)  "<IPM_Line01_C3>"
  Bus Selector2/5 -> Embedded MATLAB Function5/6(IPM_Line_C3)  "<IPM_Line03_C3>"
  Embedded MATLAB Function6/1(line_data) -> Switch3/3
  Bus Selector10/4 -> Embedded MATLAB Function9/3(IPM_Line_C1), Embedded MATLAB Function2/3(IPM_Line_C1)  "<IPM_Line01_C1>"
  Embedded MATLAB Function5/2(line_data) -> Switch3/1
  Demux/3 -> Bus Creator/3  "IPM_Line_C2"
  Bus Selector2/4 -> Embedded MATLAB Function5/5(IPM_Line_C2)  "<IPM_Line03_C2>"
  Demux1/3 -> Bus Creator1/3  "IPM_Line_C2"
  Bus Selector10/2 -> Embedded MATLAB Function6/3(IPM_Line_type), Embedded MATLAB Function5/1(IPM_Line_type)  "<IPM_Line01_Type>"
  IPM_Line_right/1 -> Bus Selector1/1
  Bus Selector10/3 -> Embedded MATLAB Function9/2(IPM_Line_C0), Embedded MATLAB Function2/2(IPM_Line_C0)  "<IPM_Line01_C0>"
  Embedded MATLAB Function1/1(line_data) -> Switch1/3
  IPM_Line_right_right/1 -> Bus Selector3/1
  Bus Selector3/5 -> Embedded MATLAB Function7/6(IPM_Line_C3)  "<IPM_Line04_C3>"
  Degrees to Radians/1 -> Divide1/1

== system ALL_JP360_DBW_V6_5_1103/CIPV1/Obstacle selection ==
  ego_lane_obstacles : Inport
  left_lane_obstacles : Inport  Port=2
  right_lane_obstacles : Inport  Port=3
  MRR_ObjID : Inport  Port=4
  MRR_ObjDistX : Inport  Port=5
  MRR_ObjDistY : Inport  Port=6
  MRR_ObjRelVelX : Inport  Port=7
  MRR_ObjRelVelY : Inport  Port=8
  MRR_ObjType : Inport  Port=9
  MRR_ObjUpdFlg : Inport  Port=10
  last_cipv : Inport  Port=11
  IPM_Obj : Inport  Port=12
  MRR_ObjFusionSig : Inport  Port=13
  MRR_ObjFusionCamID : Inport  Port=14
  Assignment : Assignment  DiagnosticForDimensions=Warning  IndexOptions=Index vector (port)  Indices=1  OutputSizes=1
  Constant : Constant  Value=200  OutDataTypeStr=single
  Constant1 : Constant  OutDataTypeStr=single
  Constant2 : Constant  Value=0  OutDataTypeStr=single
  Constant3 : Constant  OutDataTypeStr=single
  Constant4 : Constant  Value=0  OutDataTypeStr=single
  Constant5 : Constant  Value=0  OutDataTypeStr=single
  Maximum : dspstat3/Maximum  operation=maximum  fcn=Value  indexBase=One  operateOver=Specified dimension  Dimension=1  InputProcessing=Columns as channels (frame based)  reset=None  roiEnable=off  roiType=Rectangles  roiPortion=Entire ROI  roiOutput=Individual statistics for each ROI  roiFlag=off  roundingMode=Floor  overflowMode=off  accumDataTypeStr=Inherit: Same as product output  accumLastDataTypeStr=Inherit: Same as product output
  Minimum : dspstat3/Minimum  operation=minimum  fcn=Value and Index  indexBase=One  operateOver=Specified dimension  Dimension=1  InputProcessing=Columns as channels (frame based)  reset=None  roiEnable=off  roiType=Rectangles  roiPortion=Entire ROI  roiOutput=Individual statistics for each ROI  roiFlag=off  roundingMode=Floor  overflowMode=off
      settings: SourceProductBaseCode=DS
  Minimum1 : dspstat3/Minimum  operation=minimum  fcn=Value and Index  indexBase=One  operateOver=Specified dimension  Dimension=1  InputProcessing=Columns as channels (frame based)  reset=None  roiEnable=off  roiType=Rectangles  roiPortion=Entire ROI  roiOutput=Individual statistics for each ROI  roiFlag=off  roundingMode=Floor  overflowMode=off
      settings: SourceProductBaseCode=DS
  Product : Product
  Subsystem : Subsystem
  Subsystem1 : Subsystem
  Switch : Switch  Criteria=u2 > Threshold  SaturateOnIntegerOverflow=off  InputSameDT=off
  Switch1 : Switch  Criteria=u2 > Threshold  SaturateOnIntegerOverflow=off  InputSameDT=off
  Switch2 : Switch  Criteria=u2 > Threshold  SaturateOnIntegerOverflow=off  InputSameDT=off
  Switch3 : Switch  Criteria=u2 ~= 0  SaturateOnIntegerOverflow=off  InputSameDT=off
  get min : Subsystem
  get min1 : Subsystem
  cipv1 : Outport
  cipv2 : Outport  Port=2
  left_obj : Outport  Port=3
  right_obj : Outport  Port=4
  wires:
  Constant/1 -> Assignment/2, Switch/3
  Product/1 -> Assignment/1, Switch/2, Switch/1, Maximum/1
  Minimum/2 -> [CIPV_index1]
  Minimum/1 -> Switch1/2
  Constant2/1 -> Switch1/3
  Constant1/1 -> Switch1/1
  [CIPV_index1] -> Assignment/3
  Assignment/1 -> Minimum1/1
  Minimum1/2 -> [CIPV_index2]
  Minimum1/1 -> Switch2/2
  Constant3/1 -> Switch2/1
  Constant4/1 -> Switch2/3
  Switch2/1 -> [CIPV2_ObjDetected]
  left_lane_obstacles/1 -> get min/1(left_lane_obstacles)
  get min/1(is_vaild) -> [left_obj_vaild]
  get min/2(idx) -> [left_obj_idx]
  MRR_ObjDistX/1 -> [MRR_ObjDistX]
  [MRR_ObjDistX] -> Product/2
  MRR_ObjID/1 -> Subsystem/1(MRR_ObjID)
  MRR_ObjDistY/1 -> Subsystem/3(MRR_ObjDistY)
  MRR_ObjRelVelX/1 -> Subsystem/4(MRR_ObjRelVelX)
  [MRR_ObjDistX] -> Subsystem/2(MRR_ObjDistX)
  MRR_ObjRelVelY/1 -> Subsystem/5(MRR_ObjRelVelY)
  MRR_ObjType/1 -> Subsystem/6(MRR_ObjType)
  [CIPV_index1] -> Subsystem/7(CIPV_index1)
  [CIPV_index2] -> Subsystem/8(CIPV_index2)
  [left_obj_idx] -> Subsystem/9(left_obj_idx)
  [right_obj_idx] -> Subsystem/10(right_obj_idx)
  MRR_ObjUpdFlg/1 -> Subsystem/11(MRR_ObjUpdFlg)
  [CIPV1_ObjDetected] -> Subsystem/12(CIPV1_ObjDetected)
  [CIPV2_ObjDetected] -> Subsystem/13(CIPV2_ObjDetected)
  [right_obj_vaild] -> Subsystem/15(right_obj_vaild)
  [left_obj_vaild] -> Subsystem/14(left_obj_vaild)
  Subsystem/2(cipv2) -> cipv2/1
  Subsystem/3(left_obj) -> left_obj/1
  Subsystem/4(right_obj) -> right_obj/1
  Subsystem1/1(out_cipv1) -> cipv1/1
  Subsystem/1(cipv1) -> Subsystem1/1(now_cipv1)
  last_cipv/1 -> Subsystem1/2(last_cipv1)
  Constant5/1 -> Switch3/3
  Switch3/1 -> [CIPV1_ObjDetected]
  Maximum/1 -> Switch3/2
  Switch1/1 -> Switch3/1
  Switch/1 -> Minimum/1
  ego_lane_obstacles/1 -> Product/1
  [MRR_ObjDistX] -> get min/2(MRR_ObjDistX)
  get min1/2(idx1) -> [right_obj_idx]
  get min1/1(is_vaild1) -> [right_obj_vaild]
  right_lane_obstacles/1 -> get min1/1(right_lane_obstacles)
  [MRR_ObjDistX] -> get min1/2(MRR_ObjDistX)
  IPM_Obj/1 -> [IPM_Obj]
  MRR_ObjFusionSig/1 -> [MRR_ObjFusionSig]
  MRR_ObjFusionCamID/1 -> [MRR_ObjFusionCamID]
  [IPM_Obj] -> Subsystem/16(IPM_Obj)
  [MRR_ObjFusionSig] -> Subsystem/17(MRR_ObjFusionSig)
  [MRR_ObjFusionCamID] -> Subsystem/18(MRR_ObjFusionCamID)
  [IPM_Obj] -> Subsystem1/3(IPM_Obj)

== system ALL_JP360_DBW_V6_5_1103/CIPV1/filter ==
  MRR_ObjDistX : Inport
  MRR_ObjDistY : Inport  Port=2
  MRR_ObjExistProb : Inport  Port=3
  MRR_ObjFusionCamID : Inport  Port=4
  MRR_ObjFusionSig : Inport  Port=5
  MRR_ObjMovingSts : Inport  Port=6
  MRR_ObjObstacleProb : Inport  Port=7
  MRR_ObjRelVelX : Inport  Port=8
  MRR_ObjRelVelY : Inport  Port=9
  MRR_ObjType : Inport  Port=10
  left_line : Inport  Port=11
  right_line : Inport  Port=12
  Ego_speed : Inport  Port=13
  IPM_objs : Inport  Port=14
  Display10 : Display
  Filter ROI objs : Subsystem
  Filter low probability objs : Subsystem
  MRR_ObjDistXDisplay : Display
  MRR_ObjDistYDisplay : Display
  MRR_ObjExistProb Display : Display
  MRR_ObjFusionCamID Display : Display
  MRR_ObjFusionSigDisplay : Display
  MRR_ObjObstacleProbDisplay : Display
  MRR_ObjRelVelXDisplay : Display
  MRR_ObjTypeDisplay : Display
  ROI_objsDisplay : Display
  Terminator : Terminator
  ego_lane_obstaclesDisplay : Display
  filter lanes : Subsystem
  filter speed : Subsystem
  filter_speed_objsDisplay : Display
  get objs width : Subsystem
  high_probability_objsDisplay : Display
  ego_lane_obstacles : Outport
  left_lane_obstacles : Outport  Port=2
  right_lane_obstacles : Outport  Port=3
  wires:
  MRR_ObjExistProb/1 -> Filter low probability objs/1(MRR_ObjExistProb), MRR_ObjExistProb Display/1
  [high_probability_objs] -> Filter ROI objs/1(last_vaild_objs)
  Filter ROI objs/1(ROI objs) -> ROI_objsDisplay/1, [ROI_objs]
  MRR_ObjRelVelX/1 -> MRR_ObjRelVelXDisplay/1, filter speed/2(MRR_ObjRelVelX)
  [ROI_objs] -> filter speed/1(last_vaild_objs)
  Ego_speed/1 -> Display10/1, filter speed/3(ego_speed)
  filter speed/1(filter speed objs) -> filter_speed_objsDisplay/1, [filter_speed_objs]
  MRR_ObjObstacleProb/1 -> MRR_ObjObstacleProbDisplay/1, Filter low probability objs/2(MRR_ObjObstacleProb)
  Filter low probability objs/1(ourtput_filtered) -> high_probability_objsDisplay/1, [high_probability_objs]
  MRR_ObjDistX/1 -> [MRR_ObjDistX]
  MRR_ObjDistY/1 -> [MRR_ObjDistY]
  [MRR_ObjDistX] -> MRR_ObjDistXDisplay/1, Filter ROI objs/2(MRR_ObjDistX)
  [MRR_ObjDistY] -> Filter ROI objs/3(MRR_ObjDistY1), MRR_ObjDistYDisplay/1
  left_line/1 -> filter lanes/1(left_line)
  right_line/1 -> filter lanes/2(right_line)
  [MRR_ObjDistY] -> filter lanes/3(MRR_ObjDistY)
  MRR_ObjRelVelY/1 -> filter lanes/4(MRR_ObjRelVelY)
  [filter_speed_objs] -> filter lanes/5(last_vaild_objs)
  MRR_ObjFusionCamID/1 -> MRR_ObjFusionCamID Display/1, get objs width/1(MRR_ObjFusionCamID)
  MRR_ObjFusionSig/1 -> MRR_ObjFusionSigDisplay/1, get objs width/2(MRR_ObjFusionSig)
  [filter_speed_objs] -> get objs width/3(last_vaild_objs)
  get objs width/1(objs_width) -> filter lanes/6(objs_width)
  MRR_ObjMovingSts/1 -> filter lanes/7(MRR_ObjMovingSts)
  filter lanes/3(ego_lane_obstacles) -> ego_lane_obstaclesDisplay/1, ego_lane_obstacles/1
  filter lanes/1(left_lane_obstacles) -> left_lane_obstacles/1
  filter lanes/2(right_lane_obstacles) -> right_lane_obstacles/1
  MRR_ObjType/1 -> [MRR_ObjType]
  [MRR_ObjType] -> MRR_ObjTypeDisplay/1, Filter low probability objs/3(MRR_ObjType)
  [MRR_ObjType] -> get objs width/4(MRR_ObjType)
  IPM_objs/1 -> Terminator/1

== system ALL_JP360_DBW_V6_5_1103/CanbusControl/Limit ==
  Input : Inport
  Input1 : Inport  Port=2
  Input2 : Inport  Port=3
  Constant : Constant  Value=300
  Constant1 : Constant  Value=0
  Constant2 : Constant  Value=2.5  OutDataTypeStr=single
  Constant3 : Constant  Value=-2.5  OutDataTypeStr=single
  Constant4 : Constant  Value=0.1
  Constant5 : Constant  Value=-4
  Switch : Switch  Criteria=u2 > Threshold  SaturateOnIntegerOverflow=off  InputSameDT=off
  Switch1 : Switch  Criteria=u2 > Threshold  Threshold=200  SaturateOnIntegerOverflow=off  InputSameDT=off
  Switch2 : Switch  Threshold=-2.5  SaturateOnIntegerOverflow=off  InputSameDT=off
  Switch3 : Switch  Threshold=2.5  SaturateOnIntegerOverflow=off  InputSameDT=off
  Switch4 : Switch  Criteria=u2 > Threshold  Threshold=-5  SaturateOnIntegerOverflow=off  InputSameDT=off
  Switch5 : Switch  Criteria=u2 > Threshold  Threshold=0.1  SaturateOnIntegerOverflow=off  InputSameDT=off
  Out1 : Outport
  Out2 : Outport  Port=2
  Out3 : Outport  Port=3
  wires:
  Switch3/1 -> Out1/1
  Input1/1 -> Switch/2, Switch/1
  Switch1/1 -> Out2/1
  Switch5/1 -> Out3/1
  Constant/1 -> Switch1/1
  Switch/1 -> Switch1/3, Switch1/2
  Constant1/1 -> Switch/3
  Constant3/1 -> Switch2/3
  Switch2/1 -> Switch3/2, Switch3/3
  Constant2/1 -> Switch3/1
  Input/1 -> Switch2/1, Switch2/2
  Constant5/1 -> Switch4/3
  Switch4/1 -> Switch5/2, Switch5/3
  Constant4/1 -> Switch5/1
  Input2/1 -> Switch4/1, Switch4/2

== system ALL_JP360_DBW_V6_5_1103/CanbusControl/Subsystem4 ==
  In1 : Inport
  Chart : Stateflow chart  TreatAsAtomicUnit=on
  data1 : Outport
  wires:
  In1/1 -> Chart/1(data)
  Chart/1(data1) -> data1/1

== system ALL_JP360_DBW_V6_5_1103/DCLC1/DCLC planner ==
  note: 0	：DCLC功能关闭
      | 10	：DCLC功能受限
      | 11	：允许左变道
      | 12	：允许右变道
      | 13	：允许左/右变道
      | 21	：左变道等待
      | 22	：左变道中
      | 23	：左变道回退
      | 24	：左变道结束
      | 31	：右变道等待
      | 32	：右变道中
      | 33	：右变道回退
      | 34	：右变道结束
  vx : Inport
  dclc_sts : Inport  Port=2
  c0 : Inport  Port=3
  C1 : Inport  Port=4
  start_position : Inport  Port=5
  lon_weight : Inport  Port=6
  lat_weight : Inport  Port=7
  change_time_weight : Inport  Port=8
  turn_request : Inport  Port=9
  Constant : Constant  Value=-0.3
  Constant1 : Constant  Commented=on  Value=0.01
  Product : Product  Inputs=3
  Product1 : Product  Commented=on  Inputs=3
  Scope : Scope
  Scope1 : Scope
  Sin : Trigonometry
  Sin1 : Trigonometry  Commented=on  Operator=cos
  Tan : Trigonometry  Operator=atan
  change lane : MATLAB Function
  error_compute : MATLAB Function  TreatAsAtomicUnit=on  SystemSampleTime=0.01
  width compute : MATLAB Function  TreatAsAtomicUnit=on
  xrr : Outport
  yrr : Outport  Port=2
  theta : Outport  Port=3
  kr : Outport  Port=4
  reach_dest : Outport  Port=5
  status : Outport  Port=6
  wires:
  error_compute/4(krr) -> kr/1  "kr"
  change lane/1(status) -> Scope1/1, width compute/2(status), status/1
  width compute/1(y) -> error_compute/2(width)
  error_compute/2(yrr) -> yrr/1  "yrr"
  error_compute/3(thetarr) -> theta/1  "theta"
  vx/1 -> Product/1, Product1/1
  error_compute/1(xrr) -> xrr/1  "xrr"
  c0/1 -> change lane/2(c0)
  start_position/1 -> error_compute/1(start_position)
  width compute/2(change_end_status) -> reach_dest/1
  change lane/2(width) -> width compute/1(u)
  Tan/1 -> Sin1/1, Sin/1, width compute/3(heading), error_compute/4(heading)
  Sin/1 -> Product/2
  Constant/1 -> Product/3
  Product/1 -> error_compute/5(diff_y)
  Sin1/1 -> Product1/2
  Constant1/1 -> Product1/3
  Product1/1 -> error_compute/6(diff_x)
  change lane/3(heading) -> Tan/1
  C1/1 -> change lane/3(c1)
  dclc_sts/1 -> change lane/1(dclc_sts), error_compute/3(status)
  change lane/4(diff_y) -> Scope/1
  turn_request/1 -> change lane/4(turn_request)
